simulink model "BLDC_MotorDrive"  (Simulink 7.9)
settings: Solver=ode4  StartTime=0.0  StopTime=1.5  FixedStep=1e-4  RelTol=1e-3
InitFcn:
  | startup_drive
values from neighbouring files (symbols this model uses):
  B = 0    [startup_drive.m]
  bw = 0.01    [startup_drive.m]
  Jeq = 152e-6    (= 0.000152)    [startup_drive.m]
  Ke = 0.1    [startup_drive.m]
  KiP = 0    [startup_drive.m]
  KiW = 300/2    (= 150)    [startup_drive.m]
  KpP = 62.8/2    (= 31.4)    [startup_drive.m]
  KpW = 0.83/2    (= 0.415)    [startup_drive.m]
  Kpwm = 12    [startup_drive.m]
  Kt = 0.1    [startup_drive.m]
  La = 5.2e-3    (= 0.0052)    [startup_drive.m]
  Ra = 2    [startup_drive.m]
undefined symbols (not defined in the file or in its folder): currentgen
settings Model: RequirementInfo="{}  %GIDa_d07f742e_1eb0_43fa_80f3_4d465b19ddf7"  Creator=Narasimha Prasad  LastModifiedBy=Narasimha Prasad  SimulationMode=accelerator

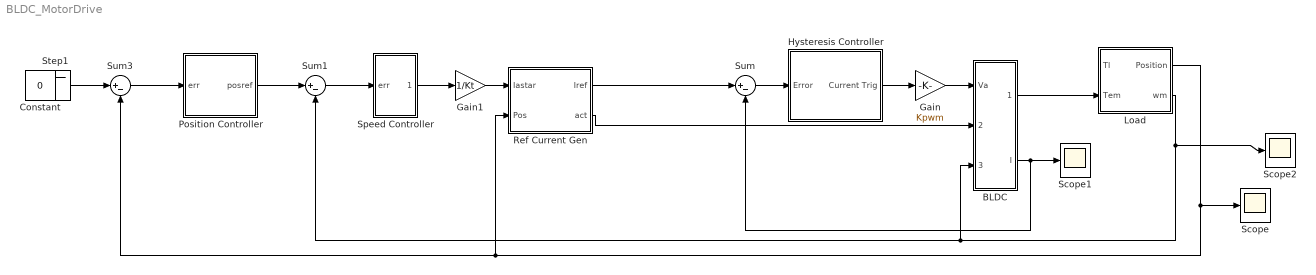
== system BLDC_MotorDrive ==
  BLDC : Subsystem
  Gain : Gain  Gain=Kpwm
  Gain1 : Gain  Gain=1/Kt
  Hysteresis Controller : Subsystem
  Load : Subsystem
  Position Controller : Subsystem
  Ref Current Gen : Subsystem
  Scope : Scope
      settings: TimeRange=0.003467476989474583  YMin=2342  YMax=2358
  Scope1 : Scope
      settings: TimeRange=0.003467476989474583  YMin=19.9986  YMax=20.0006
  Scope2 : Scope
      settings: TimeRange=0.003467476989474583  YMin=2460  YMax=2545  SaveName=ScopeData2
  Speed Controller : Subsystem
  Step1 : Step  Time=0.5  After=10  SampleTime=0
  Sum : Sum  Inputs=|+-  RndMeth=Convergent
  Sum1 : Sum  Inputs=|+-
  Sum3 : Sum  Inputs=|+-
  Constant : Constant  IOType=siggen  Value=0
  wires:
  BLDC/1(Tem) -> Load/2(Tem)
  Sum/1 -> Hysteresis Controller/1(Error)
  Hysteresis Controller/1(Current Trig) -> Gain/1
  Gain/1 -> BLDC/1(Va)
  BLDC/2(I) -> Sum/2, Scope1/1
  Ref Current Gen/2(act) -> BLDC/2(act)
  Ref Current Gen/1(Iref) -> Sum/1
  Load/1(Position) -> Scope/1, Ref Current Gen/2(Pos), Sum3/2
  Gain1/1 -> Ref Current Gen/1(Iastar)
  Load/2(wm) -> BLDC/3(wm), Sum1/2, Scope2/1
  Speed Controller/1(wref) -> Gain1/1
  Sum1/1 -> Speed Controller/1(err)
  Position Controller/1(posref) -> Sum1/1
  Sum3/1 -> Position Controller/1(err)
  Step1/1 -> Sum3/1

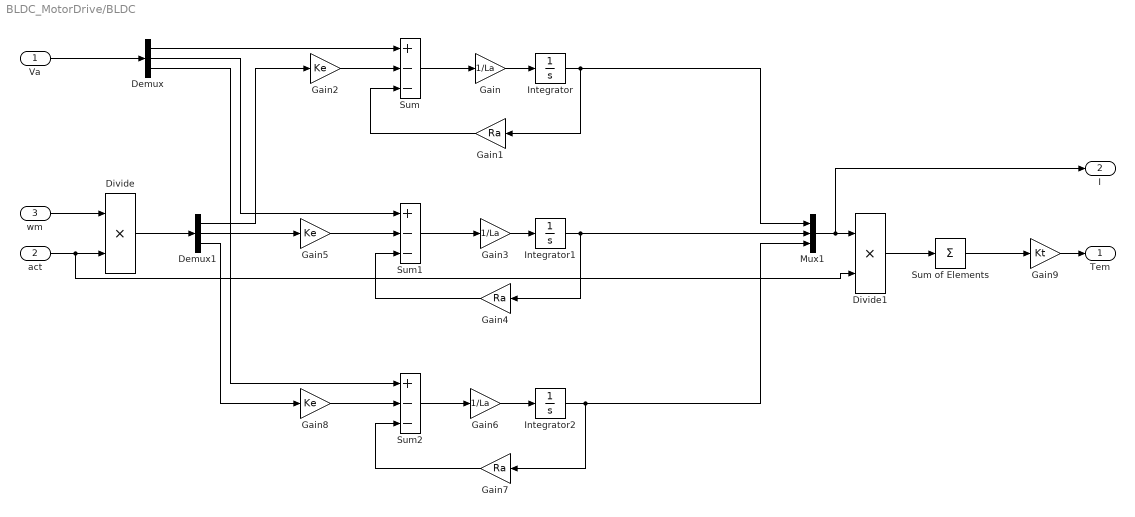
== system BLDC_MotorDrive/BLDC ==
  Va : Inport
  act : Inport  Port=2
  wm : Inport  Port=3
  Demux : Demux  Outputs=3
  Demux1 : Demux  Outputs=3
  Divide : Product  Inputs=**
  Divide1 : Product  Inputs=**
  Gain : Gain  Gain=1/La
  Gain1 : Gain  Gain=Ra
  Gain2 : Gain  Gain=Ke
  Gain3 : Gain  Gain=1/La
  Gain4 : Gain  Gain=Ra
  Gain5 : Gain  Gain=Ke
  Gain6 : Gain  Gain=1/La
  Gain7 : Gain  Gain=Ra
  Gain8 : Gain  Gain=Ke
  Gain9 : Gain  Gain=Kt
  Integrator : Integrator
  Integrator1 : Integrator
  Integrator2 : Integrator
  Mux1 : Mux  Inputs=3
  Sum : Sum  Inputs=+--
  Sum of Elements : Sum  Inputs=+
  Sum1 : Sum  Inputs=+--
  Sum2 : Sum  Inputs=+--
  Tem : Outport
  I : Outport  Port=2
  wires:
  Sum/1 -> Gain/1
  Gain/1 -> Integrator/1
  Gain1/1 -> Sum/3
  Gain2/1 -> Sum/2
  Sum1/1 -> Gain3/1
  Gain3/1 -> Integrator1/1
  Gain4/1 -> Sum1/3
  Gain5/1 -> Sum1/2
  Sum2/1 -> Gain6/1
  Gain6/1 -> Integrator2/1
  Gain7/1 -> Sum2/3
  Gain8/1 -> Sum2/2
  Demux/1 -> Sum/1
  Demux/2 -> Sum1/1
  Demux/3 -> Sum2/1
  Integrator/1 -> Gain1/1, Mux1/1
  Integrator1/1 -> Gain4/1, Mux1/2
  Integrator2/1 -> Gain7/1, Mux1/3
  Gain9/1 -> Tem/1
  wm/1 -> Divide/1
  act/1 -> Divide/2, Divide1/2
  Divide/1 -> Demux1/1
  Demux1/1 -> Gain2/1
  Demux1/2 -> Gain5/1
  Demux1/3 -> Gain8/1
  Va/1 -> Demux/1
  Mux1/1 -> Divide1/1, I/1
  Divide1/1 -> Sum of Elements/1
  Sum of Elements/1 -> Gain9/1

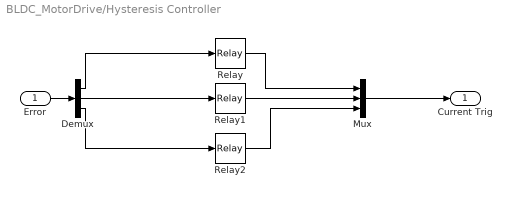
== system BLDC_MotorDrive/Hysteresis Controller ==
  Error : Inport
  Demux : Demux  Outputs=3
  Mux : Mux  Inputs=3
  Relay : Relay  RequirementInfo="{'linktype_rmi_simulink' '$ModelName$' ':112' 'true' '/Hysteresis Controller/Relay1  (Relay)' '' } %GIDa_fdfbe1ad_7fcb_4c48_adad_d014d0a27ebc"  OnSwitchValue=bw  OffSwitchValue=-bw  OnOutputValue=OnLim  OffOutputValue=OffLim  ZeroCross=off
  Relay1 : Relay  RequirementInfo={} %GIDa_6cb4c59d_d971_44c6_bd96_ecb9e994547a  OnSwitchValue=bw  OffSwitchValue=-bw  OnOutputValue=OnLim  OffOutputValue=OffLim
  Relay2 : Relay  RequirementInfo="{}  %GIDa_6bc164ec_455d_4c9c_9bc4_b9a98dcd72e8"  OnSwitchValue=bw  OffSwitchValue=-bw  OnOutputValue=OnLim  OffOutputValue=OffLim  ZeroCross=off
  Current Trig : Outport
  wires:
  Demux/1 -> Relay/1
  Demux/2 -> Relay1/1
  Demux/3 -> Relay2/1
  Relay/1 -> Mux/1
  Relay1/1 -> Mux/2
  Relay2/1 -> Mux/3
  Error/1 -> Demux/1
  Mux/1 -> Current Trig/1

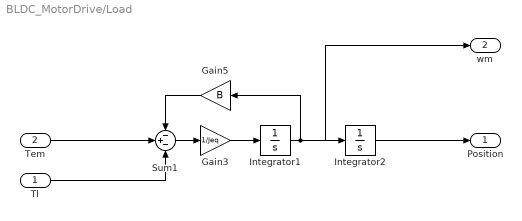
== system BLDC_MotorDrive/Load ==
  Tl : Inport
  Tem : Inport  Port=2
  Gain3 : Gain  Gain=1/Jeq
  Gain5 : Gain  Gain=B
  Integrator1 : Integrator
  Integrator2 : Integrator
  Sum1 : Sum  Inputs=-+-
  Position : Outport
  wm : Outport  Port=2
  wires:
  Sum1/1 -> Gain3/1
  Gain3/1 -> Integrator1/1
  Integrator1/1 -> Gain5/1, wm/1, Integrator2/1
  Tem/1 -> Sum1/2
  Tl/1 -> Sum1/3
  Gain5/1 -> Sum1/1
  Integrator2/1 -> Position/1

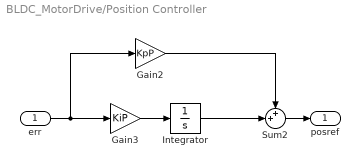
== system BLDC_MotorDrive/Position Controller ==
  err : Inport
  Gain2 : Gain  Gain=KpP
  Gain3 : Gain  Gain=KiP
  Integrator : Integrator
  Sum2 : Sum  Inputs=++|
  posref : Outport
  wires:
  Gain3/1 -> Integrator/1
  Gain2/1 -> Sum2/1
  Integrator/1 -> Sum2/2
  err/1 -> Gain3/1, Gain2/1
  Sum2/1 -> posref/1

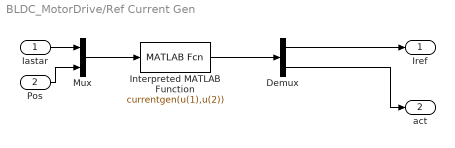
== system BLDC_MotorDrive/Ref Current Gen ==
  Iastar : Inport
  Pos : Inport  Port=2
  Demux : Demux  Outputs=2
  Interpreted MATLAB Function : MATLABFcn  MATLABFcn=currentgen(u(1),u(2))  Output1D=off
  Mux : Mux  Inputs=2
  Iref : Outport
  act : Outport  Port=2
  wires:
  Interpreted MATLAB Function/1 -> Demux/1
  Iastar/1 -> Mux/1
  Demux/1 -> Iref/1
  Demux/2 -> act/1
  Pos/1 -> Mux/2
  Mux/1 -> Interpreted MATLAB Function/1

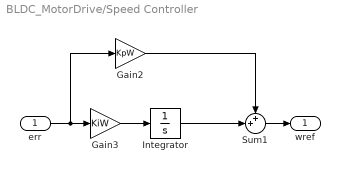
== system BLDC_MotorDrive/Speed Controller ==
  err : Inport
  Gain2 : Gain  Gain=KpW
  Gain3 : Gain  Gain=KiW
  Integrator : Integrator
  Sum1 : Sum  Inputs=++|
  wref : Outport
  wires:
  Integrator/1 -> Sum1/2
  Gain2/1 -> Sum1/1
  Gain3/1 -> Integrator/1
  err/1 -> Gain2/1, Gain3/1
  Sum1/1 -> wref/1
